simulink model "DSP_2_demo_RAM"  (R2024b)
settings: Solver=VariableStepAuto  StartTime=0.0  StopTime=10.0  RelTol=1e-3
libraries: hdlsllib x3, simulink x1
settings Model: Creator=amitk  LastModifiedBy=amitk

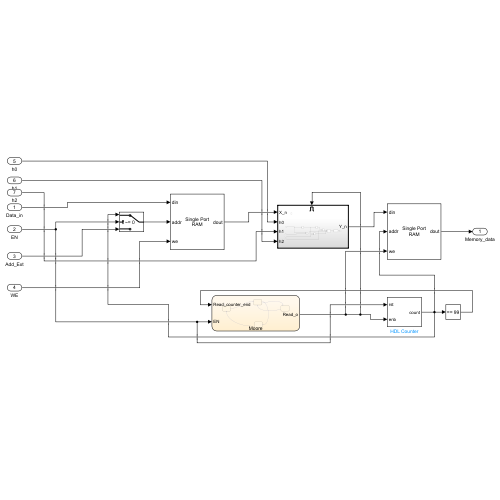
[thumbnail: Simulink's stored preview of the top-level diagram]
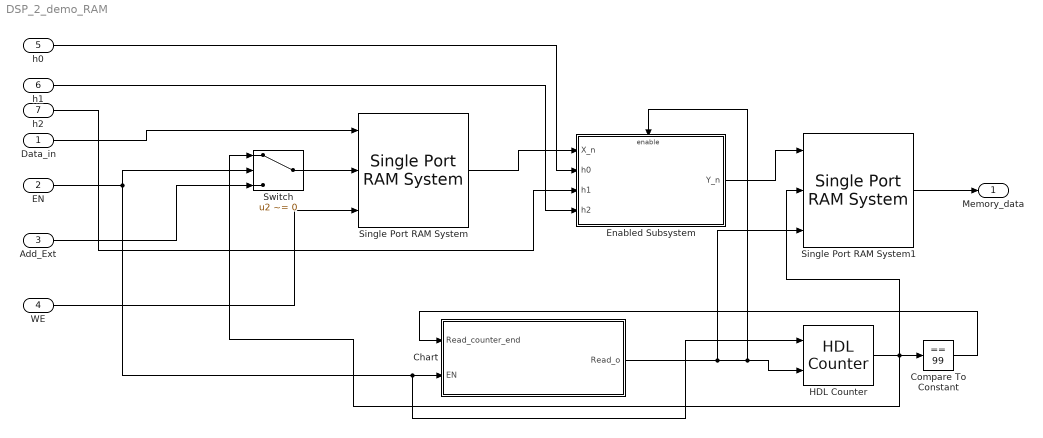
== system DSP_2_demo_RAM ==
  Data_in : Inport  OutDataTypeStr=fixdt(1,8,6)
      settings: SignalType=complex
  EN : Inport  Port=2  OutDataTypeStr=boolean
  Add_Ext : Inport  Port=3  OutDataTypeStr=uint8
      settings: SignalType=complex
  WE : Inport  Port=4  OutDataTypeStr=boolean
  h0 : Inport  Port=5  OutDataTypeStr=fixdt(1,6,4)
      settings: SignalType=complex
  h1 : Inport  Port=6  OutDataTypeStr=fixdt(1,6,4)
      settings: SignalType=complex
  h2 : Inport  Port=7  OutDataTypeStr=fixdt(1,6,4)
      settings: SignalType=complex
  Chart : Stateflow chart  TreatAsAtomicUnit=on
  Compare To Constant : simulink/Logic and Bit Operations/Compare To Constant  relop===  const=99  OutDataTypeStr=boolean
  Enabled Subsystem : Subsystem  TreatAsAtomicUnit=on
  HDL Counter : hdlsllib/Sources/HDL Counter  CountType=Count limited  CountInit=0  CountStep=1  CountMax=1000  CountFromType=Initial value  CountFrom=0  CountResetPort=on  CountLoadPort=off  CountEnbPort=on  CountDirPort=off  CountHitOutputPort=off  CountDataType=Unsigned  CountWordLen=12  CountFracLen=0  CountSampTime=1
  Single Port RAM System : hdlsllib/HDL RAMs/Single Port RAM System  RAMType=Single port  AsyncRead=off  WriteOutputValue=New data  RAMInitialValue=0  allowBusInputs=off  WritesHaveOutput=on  NumReads=0  NumWrites=1  SimulateUsing=Code generation  ModelRAMDelay=on
  Single Port RAM System1 : hdlsllib/HDL RAMs/Single Port RAM System  RAMType=Single port  AsyncRead=off  WriteOutputValue=New data  RAMInitialValue=0  allowBusInputs=off  WritesHaveOutput=on  NumReads=0  NumWrites=1  SimulateUsing=Code generation  ModelRAMDelay=on
  Switch : Switch  Criteria=u2 ~= 0  SaturateOnIntegerOverflow=off  InputSameDT=off
  Memory_data : Outport
  wires:
  Data_in/1 -> Single Port RAM System/1
  EN/1 -> Switch/2, HDL Counter/1, Chart/2(EN)
  Switch/1 -> Single Port RAM System/2
  Add_Ext/1 -> Switch/3
  HDL Counter/1 -> Single Port RAM System1/2, Switch/1, Compare To Constant/1
  WE/1 -> Single Port RAM System/3
  Single Port RAM System/1 -> Enabled Subsystem/1(X_n)
  Chart/1(Read_o) -> Single Port RAM System1/3, Enabled Subsystem/Enable, HDL Counter/2
  h0/1 -> Enabled Subsystem/2(h0)
  h1/1 -> Enabled Subsystem/4(h2)
  h2/1 -> Enabled Subsystem/3(h1)
  Compare To Constant/1 -> Chart/1(Read_counter_end)
  Enabled Subsystem/1(Y_n) -> Single Port RAM System1/1
  Single Port RAM System1/1 -> Memory_data/1

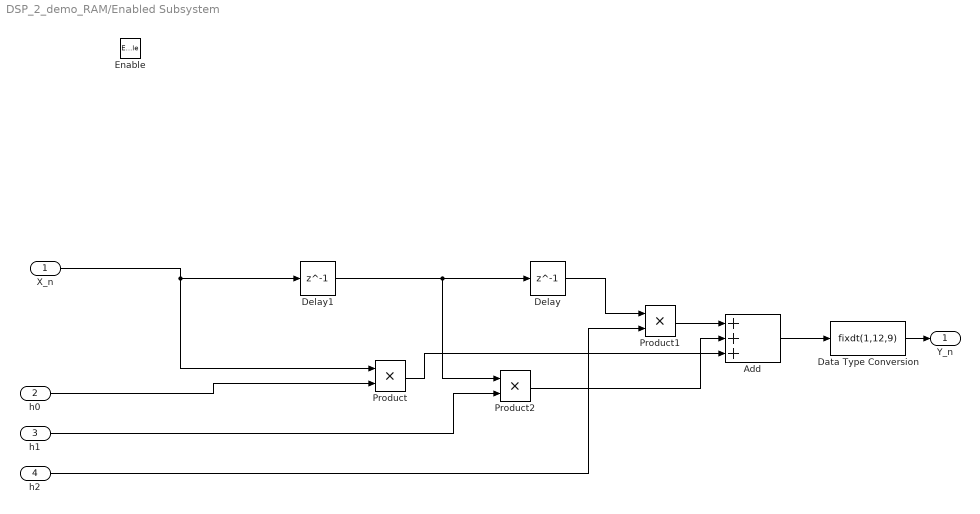
== system DSP_2_demo_RAM/Enabled Subsystem ==
  X_n : Inport  OutDataTypeStr=fixdt(1,8,6)
      settings: SignalType=complex
  h0 : Inport  Port=2  OutDataTypeStr=fixdt(1,6,4)
      settings: SignalType=complex
  h1 : Inport  Port=3  OutDataTypeStr=fixdt(1,6,4)
      settings: SignalType=complex
  h2 : Inport  Port=4  OutDataTypeStr=fixdt(1,6,4)
      settings: SignalType=complex
  Enable : EnablePort
  Add : Sum  Inputs=+++
  Data Type Conversion : DataTypeConversion  OutDataTypeStr=fixdt(1,12,9)  SaturateOnIntegerOverflow=off  RndMeth=Floor
  Delay : Delay  DelayLength=1  InitialCondition=0
  Delay1 : Delay  DelayLength=1  InitialCondition=0
  Product : Product
  Product1 : Product
  Product2 : Product
  Y_n : Outport  VectorParamsAs1DForOutWhenUnconnected=off
  wires:
  Product/1 -> Add/3
  Add/1 -> Data Type Conversion/1
  X_n/1 -> Product/1, Delay1/1
  h2/1 -> Product1/2
  Product1/1 -> Add/1
  Delay1/1 -> Product2/1, Delay/1
  Delay/1 -> Product1/1
  Data Type Conversion/1 -> Y_n/1
  h1/1 -> Product2/2
  h0/1 -> Product/2
  Product2/1 -> Add/2

== stateflow chart DSP_2_demo_RAM/Chart ==
  settings: stateMachineType=MOORE_MACHINE  executeAtInitialization=1
  state Read
    Read_o = true
  state Reset
    Read_o = false
  state Buf_state
    Read_o = false
  state Final_inter
    Read_o = false
  Reset -> Read : [EN ==1]
  Read -> Buf_state [order 1] : [Read_counter_end ==0]
  Read -> Final_inter [order 2] : [Read_counter_end ==1]
  (default) -> Reset
  Buf_state -> Read
  Final_inter -> Reset
  data: Read_counter_end input; Read_o output; EN input
